simulink model "B747_mpc_ss_du"  (Simulink 8.9)
settings: Solver=ode4  StartTime=0.0  StopTime=10  FixedStep=0.001  RelTol=1e-3
values from neighbouring files (symbols this model uses):
  Ac = [0  wr 0 ... (first row only)    [MatrizesDeEstadoSmallSize.m]    (also in mpc_ss_du_mimo.m; parametrosSmallSizeFunc.m = Ac(1,1))
  Bc = -eye(3)    [MatrizesDeEstadoSmallSize.m]    (also in mpc_ss_du_mimo.m; parametrosSmallSizeFunc.m = Bc(1,1))
  C = eye(3)    [MatrizesDeEstadoSmallSize.m]    (also in mpc_ss_du_mimo.m; parametrosSmallSizeFunc.m = [1])
  T = 0.005    [MatrizesDeEstadoSmallSize.m]    (also in SmallSizeDynamicEq.m = (1/2)*m*Vcm_quad + (1/2)*Icm*w^2; deriveRobotDynamicEquations.m = (1/2) * m * (vcm' * vcm) + (1/2) * Icm * (w' * w); deriveRobotDynamicEquations_SimulinkBlock.m = (1/2) * m * (vcm' * vcm) + (1/2) * Icm * (w' * w); mpc_ss_du_mimo.m)
undefined symbols (not defined in the file or in its folder): A, B
settings Model: Creator=Kawakami  LastModifiedBy=Pichau
settings DataIOCC: SignalLoggingName=sigsOut
settings OptimizationCC: BooleanDataType=off  ExpressionDepthLimit=2147483647
settings DebuggingCC: SaveWithParameterizedLinksMsg=none  SignalResolutionControl=TryResolveAllWithWarning  MultiTaskDSMMsg=warning  MultiTaskCondExecSysMsg=none
settings HardwareCC: TargetUnknown=on

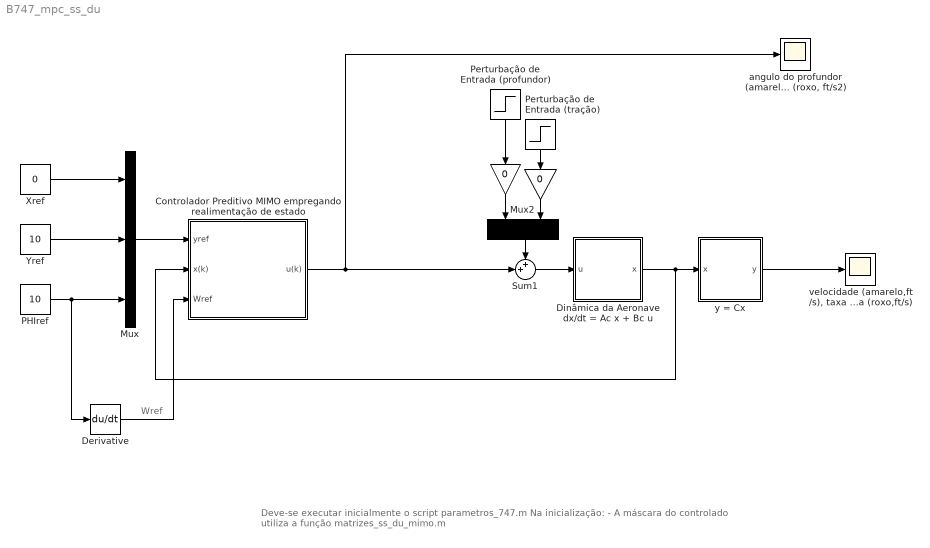
== system B747_mpc_ss_du ==
  note: Wref
  note: Deve-se executar inicialmente o script parametros_747.m
      |
      | Na inicialização:
      | - A máscara do controlado utiliza a função matrizes_ss_du_mimo.m
  " " : Gain  Gain=0
  "  " : Gain  Gain=0
  Controlador Preditivo MIMO empregando realimentação de estado : Subsystem  mask{rho=[1;1], mu=[1;1], N=10, M=5, A=A, B=B, C=C, T=T}
      mask prompts: rho "Pesos dos controles rho (p x 1)"; mu "Pesos das saídas mu (q x 1)"; N "Horizonte de Predição (N)"; M "Horizonte de Controle (M)"; A "Matriz A (n x n)"; B "Matriz B (n x p)"; C "Matriz C (q x n)"; T "Periodo de amostragem"
      mask init:
      | p = length(rho);
      | q = length(mu);
      | n = q;
  Derivative : Derivative
  Dinâmica da Aeronave dx/dt = Ac x + Bc u : Subsystem
  Mux : Mux  Inputs=3
  Mux2 : Mux  Inputs=2
  PHIref : Constant  Value=10
  Perturbação de Entrada (profundor) : Step  Time=4  After=2  SampleTime=0
  Perturbação de Entrada (tração) : Step  Time=4  After=2  SampleTime=0
  Sum1 : Sum  Inputs=++|  SaturateOnIntegerOverflow=on
  Xref : Constant  Value=0
  Yref : Constant  Value=10
  "angulo do profundor (amarelo, crad) tração específica (roxo, ft/s2)" : Scope
  "velocidade (amarelo,ft/s), taxa de subida (roxo,ft/s)" : Scope
  y = Cx : Subsystem
  wires:
  Controlador Preditivo MIMO empregando realimentação de estado/1(u(k)) -> "angulo do profundor (amarelo, crad) tração específica (roxo, ft/s2)"/1, Sum1/2
  Dinâmica da Aeronave dx/dt = Ac x + Bc u/1(x) -> y = Cx/1(x), Controlador Preditivo MIMO empregando realimentação de estado/2(x(k))
  Mux/1 -> Controlador Preditivo MIMO empregando realimentação de estado/1(yref)
  Xref/1 -> Mux/1
  Yref/1 -> Mux/2
  Sum1/1 -> Dinâmica da Aeronave dx/dt = Ac x + Bc u/1(u)
  y = Cx/1(y) -> "velocidade (amarelo,ft/s), taxa de subida (roxo,ft/s)"/1
  Mux2/1 -> Sum1/1
  Perturbação de Entrada (profundor)/1 -> "  "/1
  Perturbação de Entrada (tração)/1 -> " "/1
  "  "/1 -> Mux2/1
  " "/1 -> Mux2/2
  PHIref/1 -> Derivative/1, Mux/3
  Derivative/1 -> Controlador Preditivo MIMO empregando realimentação de estado/3(Wref)

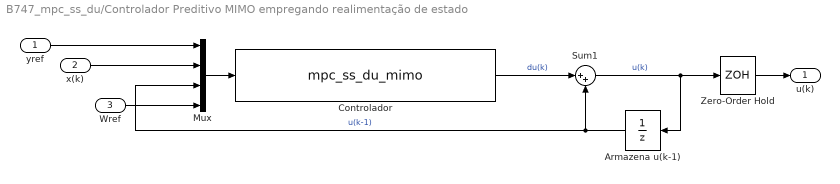
== system B747_mpc_ss_du/Controlador Preditivo MIMO empregando realimentação de estado ==
  yref : Inport
  x(k) : Inport  Port=2
  Wref : Inport  Port=3
  Armazena u(k-1) : UnitDelay  SampleTime=T
  Controlador : S-Function  FunctionName=mpc_ss_du_mimo  Parameters=p,q,n,N,T  SFunctionDeploymentMode=off  EnableBusSupport=off
  Mux : Mux
  Sum1 : Sum  Inputs=|++  SaturateOnIntegerOverflow=on  InputSameDT=on  OutDataTypeStr=Inherit: Same as first input
  Zero-Order Hold : ZeroOrderHold  SampleTime=T
  u(k) : Outport
  wires:
  Mux/1 -> Controlador/1
  Zero-Order Hold/1 -> u(k)/1
  x(k)/1 -> Mux/2
  yref/1 -> Mux/1
  Sum1/1 -> Zero-Order Hold/1, Armazena u(k-1)/1  "u(k)"
  Armazena u(k-1)/1 -> Sum1/2, Mux/3  "u(k-1)"
  Controlador/1 -> Sum1/1  "du(k)"
  Wref/1 -> Mux/4

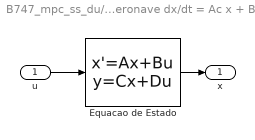
== system B747_mpc_ss_du/Dinâmica da Aeronave dx/dt = Ac x + Bc u ==
  u : Inport
  Equacao de Estado : StateSpace  A=Ac  B=Bc  C=eye(size(A,1),size(A,1))  D=zeros(size(A,1),size(B,2))  X0=zeros(size(A,1),1)
  x : Outport
  wires:
  u/1 -> Equacao de Estado/1
  Equacao de Estado/1 -> x/1

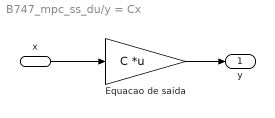
== system B747_mpc_ss_du/y = Cx ==
  x : Inport
  Equacao de saida : Gain  Gain=C  Multiplication=Matrix(K*u)  SaturateOnIntegerOverflow=on  OutDataTypeStr=Inherit: Same as input  ParamDataTypeStr=Inherit: Same as input
  y : Outport
  wires:
  x/1 -> Equacao de saida/1
  Equacao de saida/1 -> y/1
